simulink model "Virtual_Engine_Dynamometer"  (R2016b)
settings: Solver=FixedStepDiscrete  StartTime=0.0  StopTime=inf  FixedStep=VirtEngDyno.tiSimnTiStep_C.Value  RelTol=1e-3  EnableMultiTasking=on
InitFcn:
  | % Call parameters initialization function
  | % run optiTruck_init_sim.m;
StopFcn:
  | %optiTruck_post_sim;
  | %optiTruck_plot_sim;
undefined symbols (not defined in the file or in its folder): dyno_data
settings Model: Creator=engin  LastModifiedBy=bunver
settings DataIOCC: SaveFormat=StructureWithTime  SaveOutput=off  DSMLogging=off  VisualizeSimOutput=off  SaveTime=off  SignalLoggingName=Results
settings OptimizationCC: BlockReduction=off  ConditionallyExecuteInputs=off  LifeSpan=inf
settings DebuggingCC: AllowSymbolicDim=off  SFUnexpectedBacktrackingDiag=warning  SFNoUnconditionalDefaultTransitionDiag=warning  SFExecutionAtInitializationDiag=none
settings ModelReferenceCC: ModelReferenceNumInstancesAllowed=Single  PropagateSignalLabelsOutOfModel=off
settings GRTTargetCC: TargetLangStandard=C89/C90 (ANSI)
settings ConfigComp: CovMetricSettings=dw  CovHtmlReporting=on  CovSaveCumulativeToWorkspaceVar=on  CovSaveSingleToWorkspaceVar=on  CovExternalEMLEnable=off

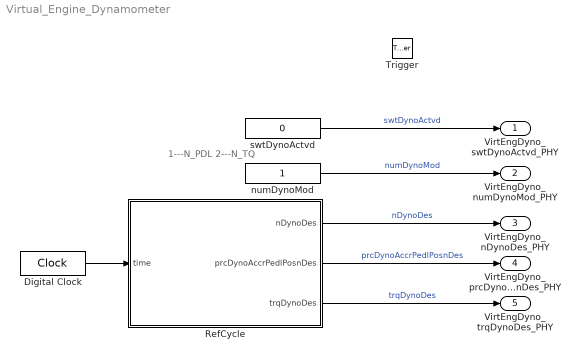
== system Virtual_Engine_Dynamometer ==
  note: 1---N_PDL
      | 2---N_TQ
  Trigger : TriggerPort  TriggerType=function-call  VariantControl=Variant  PortDimensions=1
  Digital Clock : DigitalClock  SampleTime=-1
  RefCycle : Subsystem
  numDynoMod : Constant  SampleTime=-1
  swtDynoActvd : Constant  Value=0  SampleTime=-1
  VirtEngDyno_swtDynoActvd_PHY : Outport
  VirtEngDyno_numDynoMod_PHY : Outport  Port=2
  VirtEngDyno_nDynoDes_PHY : Outport  Port=3
  VirtEngDyno_prcDynoAccrPedlPosnDes_PHY : Outport  Port=4
  VirtEngDyno_trqDynoDes_PHY : Outport  Port=5
  wires:
  Digital Clock/1 -> RefCycle/1(time)
  swtDynoActvd/1 -> VirtEngDyno_swtDynoActvd_PHY/1  "swtDynoActvd"
  numDynoMod/1 -> VirtEngDyno_numDynoMod_PHY/1  "numDynoMod"
  RefCycle/1(nDynoDes) -> VirtEngDyno_nDynoDes_PHY/1  "nDynoDes"
  RefCycle/2(prcDynoAccrPedlPosnDes) -> VirtEngDyno_prcDynoAccrPedlPosnDes_PHY/1  "prcDynoAccrPedlPosnDes"
  RefCycle/3(trqDynoDes) -> VirtEngDyno_trqDynoDes_PHY/1  "trqDynoDes"

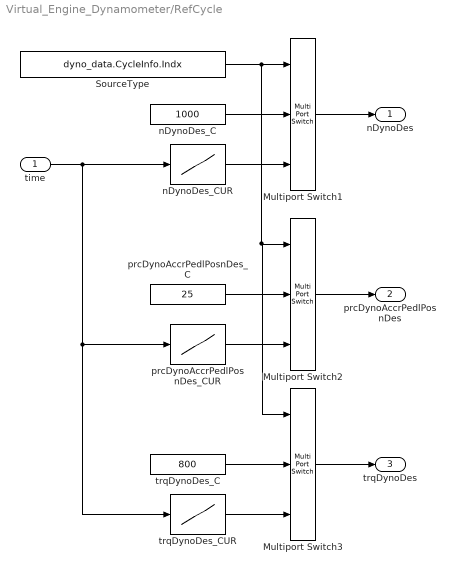
== system Virtual_Engine_Dynamometer/RefCycle ==
  time : Inport
  Multiport Switch1 : MultiPortSwitch  DataPortOrder=Zero-based contiguous  Inputs=2
  Multiport Switch2 : MultiPortSwitch  DataPortOrder=Zero-based contiguous  Inputs=2
  Multiport Switch3 : MultiPortSwitch  DataPortOrder=Zero-based contiguous  Inputs=2
  SourceType : Constant  Value=dyno_data.CycleInfo.Indx  SampleTime=-1
  nDynoDes_C : Constant  Value=1000  SampleTime=-1
  nDynoDes_CUR : Lookup_n-D  NumberOfTableDimensions=1  BreakpointsForDimension1=dyno_data.CycleInfo.Time  Table=dyno_data.CycleInfo.EngSpeed  ExtrapMethod=Clip  UseLastTableValue=on  InternalRulePriority=Speed  RndMeth=Simplest  InputSameDT=on
  prcDynoAccrPedlPosnDes_C : Constant  Value=25  SampleTime=-1
  prcDynoAccrPedlPosnDes_CUR : Lookup_n-D  NumberOfTableDimensions=1  BreakpointsForDimension1=dyno_data.CycleInfo.Time  Table=dyno_data.CycleInfo.AccrPedlPosn  ExtrapMethod=Clip  UseLastTableValue=on  InternalRulePriority=Speed  RndMeth=Simplest  InputSameDT=on
  trqDynoDes_C : Constant  Value=800  SampleTime=-1
  trqDynoDes_CUR : Lookup_n-D  NumberOfTableDimensions=1  BreakpointsForDimension1=dyno_data.CycleInfo.Time  Table=dyno_data.CycleInfo.EngTorque  ExtrapMethod=Clip  UseLastTableValue=on  InternalRulePriority=Speed  RndMeth=Simplest  InputSameDT=on
  nDynoDes : Outport
  prcDynoAccrPedlPosnDes : Outport  Port=2
  trqDynoDes : Outport  Port=3
  wires:
  SourceType/1 -> Multiport Switch3/1, Multiport Switch2/1, Multiport Switch1/1
  nDynoDes_CUR/1 -> Multiport Switch1/3
  nDynoDes_C/1 -> Multiport Switch1/2
  Multiport Switch1/1 -> nDynoDes/1
  Multiport Switch2/1 -> prcDynoAccrPedlPosnDes/1
  Multiport Switch3/1 -> trqDynoDes/1
  prcDynoAccrPedlPosnDes_C/1 -> Multiport Switch2/2
  prcDynoAccrPedlPosnDes_CUR/1 -> Multiport Switch2/3
  time/1 -> trqDynoDes_CUR/1, prcDynoAccrPedlPosnDes_CUR/1, nDynoDes_CUR/1
  trqDynoDes_C/1 -> Multiport Switch3/2
  trqDynoDes_CUR/1 -> Multiport Switch3/3
